simulink model "model_parent_phone"  (R2022a)
settings: Solver=FixedStepAuto  StartTime=0.0  StopTime=inf  RelTol=1e-3
undefined symbols (not defined in the file): Data_Display, Data_Display1, Data_Display2, Data_Display3, map_image, merged
libraries: androiduilib x5, androidcommunicationlib x5, androidaudiovideolib x2
settings Model: Creator=aditya_mangla  LastModifiedBy=aditya_mangla
settings OptimizationCC: EnhancedBackFolding=on  PassReuseOutputArgsAs=Individual arguments  ZeroExternalMemoryAtStartup=off  ZeroInternalMemoryAtStartup=off  MaxStackSize=64  OptimizeBlockOrder=speed  DifferentSizesBufferReuse=on  OptimizationCustomize=off  EfficientTunableParamExpr=on
settings DebuggingCC: ParameterTunabilityLossMsg=error
settings HardwareCC: ProdBitPerPointer=32  ProdBitPerSizeT=32  ProdBitPerPtrDiffT=32  ProdLargestAtomicInteger=Long  ProdLargestAtomicFloat=Double  ProdWordSize=32  ProdHWDeviceType=ARM Compatible->ARM Cortex  UseEmbeddedCoderFeatures=off  UseSimulinkCoderFeatures=off
settings SFSimCC: MATLABDynamicMemAlloc=off
settings RTWCC: SystemTargetFile=ert.tlc  HardwareBoard=Android Device  TLCOptions="-aInlineSetEventsForThisBaseRateFcn=TLC_FALSE -aSuppressMultiTaskScheduler=TLC_FALSE  -aRateBasedStepFcn=0"  TemplateMakefile=ert_default_tmf  RTWVerbose=off  Toolchain=Android SDK/NDK Tools
settings CodeAppCC: ForceParamTrailComments=on  IgnoreCustomStorageClasses=off  OperatorAnnotations=on  SimulinkDataObjDesc=on  SFDataObjDesc=on  InsertBlockDesc=on
settings ERTTargetCC: SupportNonInlinedSFcns=on

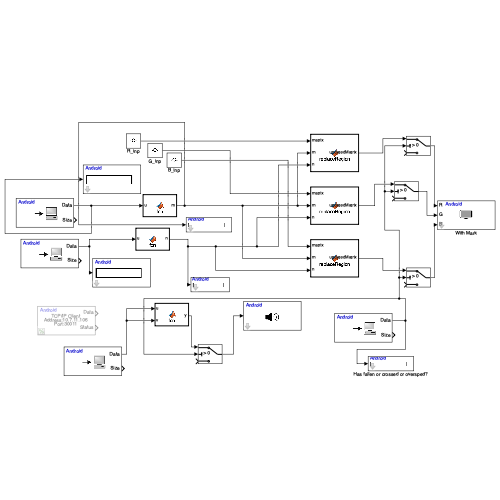
[thumbnail: Simulink's stored preview of the top-level diagram]
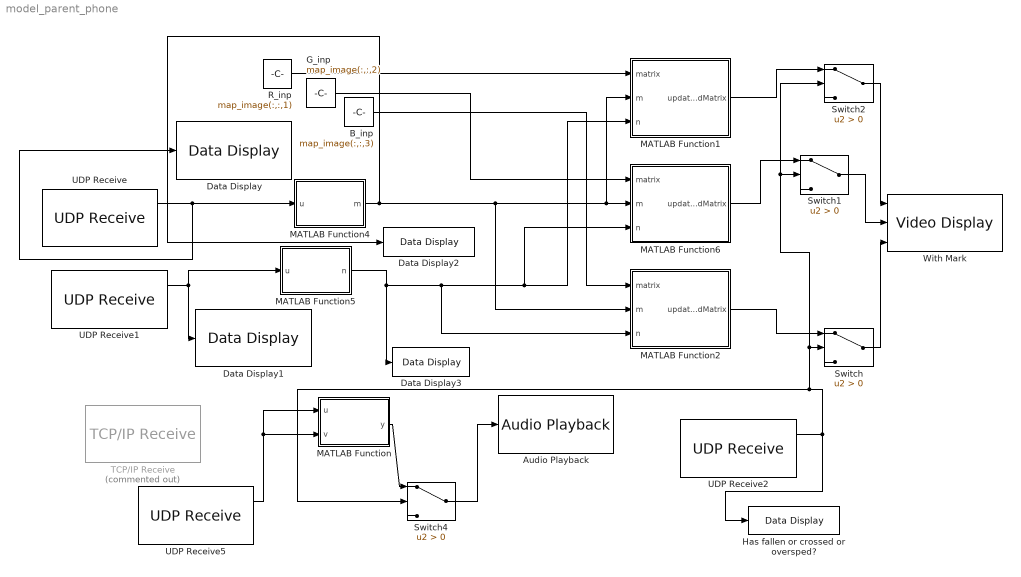
== system model_parent_phone ==
  Audio Playback : androidaudiovideolib/Audio Playback  SampleFreq=24000  AudioSamplingFreq=24000  SampleTime=0.1  DeviceStr=0  QueueDuration=0  BlockPlatform=Android
      settings: SourceProductBaseCode=ANDROID
  B_inp : Constant  Value=map_image(:,:,3)  VectorParams1D=off  OutDataTypeStr=uint8
  Data Display : androiduilib/Data Display  DataDisplayId=merged/Data_Display  Format=Float  Precision=6  SimulateUsing=Code generation  blockPlatform=Android
      settings: SourceProductBaseCode=ANDROID
  Data Display1 : androiduilib/Data Display  DataDisplayId=merged/Data_Display1  Format=Float  Precision=6  SimulateUsing=Code generation  blockPlatform=Android
      settings: SourceProductBaseCode=ANDROID
  Data Display2 : androiduilib/Data Display  DataDisplayId=merged/Data_Display2  Format=Float  Precision=6  SimulateUsing=Code generation  blockPlatform=Android
      settings: SourceProductBaseCode=ANDROID
  Data Display3 : androiduilib/Data Display  DataDisplayId=merged/Data_Display3  Format=Float  Precision=6  SimulateUsing=Code generation  blockPlatform=Android
      settings: SourceProductBaseCode=ANDROID
  G_inp : Constant  Value=map_image(:,:,2)  VectorParams1D=off  OutDataTypeStr=uint8
  Has fallen or crossed or oversped? : androiduilib/Data Display  DataDisplayId=merged/Has_fallen_or_crossed_or_oversped?  Format=Float  Precision=6  SimulateUsing=Code generation  blockPlatform=Android
      settings: SourceProductBaseCode=ANDROID
  MATLAB Function : MATLAB Function  TreatAsAtomicUnit=on
  MATLAB Function1 : MATLAB Function  TreatAsAtomicUnit=on
  MATLAB Function2 : MATLAB Function  TreatAsAtomicUnit=on
  MATLAB Function4 : MATLAB Function  TreatAsAtomicUnit=on
  MATLAB Function5 : MATLAB Function  TreatAsAtomicUnit=on
  MATLAB Function6 : MATLAB Function  TreatAsAtomicUnit=on
  R_inp : Constant  Value=map_image(:,:,1)  VectorParams1D=off  OutDataTypeStr=uint8
  Switch : Switch  Criteria=u2 > Threshold  SaturateOnIntegerOverflow=off  InputSameDT=off
  Switch1 : Switch  Criteria=u2 > Threshold  SaturateOnIntegerOverflow=off  InputSameDT=off
  Switch2 : Switch  Criteria=u2 > Threshold  SaturateOnIntegerOverflow=off  InputSameDT=off
  Switch4 : Switch  Criteria=u2 > Threshold  OutDataTypeStr=int16  SaturateOnIntegerOverflow=off  InputSameDT=off
  TCP/IP Receive : androidcommunicationlib/TCP//IP Receive  Commented=on  TCPReceiveId=Map_display/TCP//IP_Receive  Mode_=Client  LocalServerPort_=25000  RemoteAddr_=10.7.11.106  RemoteServerPort_=30011  DataType_=int16  DataSize_=2400  SampleTime_=0.1  ClientPortBindingSelection_=off  ClientPortToBind_=35000  BlockingMode_=off  BlockTimeout_=0.1
      settings: SourceProductBaseCode=ANDROID
  UDP Receive : androidcommunicationlib/UDP Receive  localURL='0.0.0.0'  localPort=30001  remoteURL='0.0.0.0'  remotePort=-1  recvBufferSize=8192  signalDatatype=double  dims=1  isVarSize=off  showBlockingTime=off  blockingTime=0  sampletime=0.1  blockPlatform=Android
      settings: SourceProductBaseCode=ANDROID
  UDP Receive1 : androidcommunicationlib/UDP Receive  localURL='0.0.0.0'  localPort=30002  remoteURL='0.0.0.0'  remotePort=-1  recvBufferSize=8192  signalDatatype=double  dims=1  isVarSize=off  showBlockingTime=off  blockingTime=0  sampletime=0.1  blockPlatform=Android
      settings: SourceProductBaseCode=ANDROID
  UDP Receive2 : androidcommunicationlib/UDP Receive  localURL='0.0.0.0'  localPort=30012  remoteURL='0.0.0.0'  remotePort=-1  recvBufferSize=8192  signalDatatype=boolean  dims=1  isVarSize=off  showBlockingTime=off  blockingTime=0  sampletime=0.1  blockPlatform=Android
      settings: SourceProductBaseCode=ANDROID
  UDP Receive5 : androidcommunicationlib/UDP Receive  localURL='0.0.0.0'  localPort=30011  remoteURL='0.0.0.0'  remotePort=-1  recvBufferSize=8192  signalDatatype=int16  dims=2400  isVarSize=off  showBlockingTime=off  blockingTime=0  sampletime=0.1  blockPlatform=Android
      settings: SourceProductBaseCode=ANDROID
  With Mark : androidaudiovideolib/Video Display  BlockPlatform=Android
      settings: SourceProductBaseCode=ANDROID
  wires:
  UDP Receive1/1 -> Data Display1/1, MATLAB Function5/1(u)
  Switch4/1 -> Audio Playback/1
  MATLAB Function1/1(updatedMatrix) -> Switch2/1
  MATLAB Function4/1(m) -> Data Display2/1, MATLAB Function1/2(m), MATLAB Function6/2(m), MATLAB Function2/2(m)
  Switch2/1 -> With Mark/1
  B_inp/1 -> MATLAB Function2/1(matrix)
  UDP Receive/1 -> Data Display/1, MATLAB Function4/1(u)
  Switch1/1 -> With Mark/2
  Switch/1 -> With Mark/3
  MATLAB Function6/1(updatedMatrix) -> Switch1/1
  R_inp/1 -> MATLAB Function1/1(matrix)
  MATLAB Function2/1(updatedMatrix) -> Switch/1
  UDP Receive5/1 -> MATLAB Function/2(v), MATLAB Function/1(u)
  G_inp/1 -> MATLAB Function6/1(matrix)
  MATLAB Function/1(y) -> Switch4/1
  MATLAB Function5/1(n) -> Data Display3/1, MATLAB Function1/3(n), MATLAB Function6/3(n), MATLAB Function2/3(n)
  UDP Receive2/1 -> Has fallen or crossed or oversped?/1, Switch4/2, Switch2/2, Switch1/2, Switch/2

== matlab function model_parent_phone/MATLAB Function1 ==
  data: updatedMatrix output; matrix input; m input; n input
function updatedMatrix = replaceRegion(matrix, m, n)
    [rows, cols] = size(matrix);
    updatedMatrix = matrix;


    rowStart = m - 7;
    rowEnd = m + 7;
    colStart = n - 7;
    colEnd = n + 7;

    rowStart = max(1, rowStart);
    rowEnd = min(rows, rowEnd);
    colStart = max(1, colStart);
    colEnd = min(cols, colEnd);

    updatedMatrix(rowStart:rowEnd, colStart:colEnd) = 255; 

end

== matlab function model_parent_phone/MATLAB Function2 ==
  data: updatedMatrix output; matrix input; m input; n input
function updatedMatrix = replaceRegion(matrix, m, n)
    [rows, cols] = size(matrix);
    updatedMatrix = matrix;


    rowStart = m - 7;
    rowEnd = m + 7;
    colStart = n - 7;
    colEnd = n + 7;

    rowStart = max(1, rowStart);
    rowEnd = min(rows, rowEnd);
    colStart = max(1, colStart);
    colEnd = min(cols, colEnd);

    updatedMatrix(rowStart:rowEnd, colStart:colEnd) = 0; 

end

== matlab function model_parent_phone/MATLAB Function4 ==
  data: u input; m output
function m = fcn(u)
    clat=5.513888888888889e-6;
    md = (23.21385-u)/clat;
    m = int16(md);

== matlab function model_parent_phone/MATLAB Function5 ==
  data: u input; n output
function n = fcn(u)
    clong= 3.42890625e-6;
    nd = (72.68525-u)/clong;
    n = int16(nd);

== matlab function model_parent_phone/MATLAB Function ==
  data: u input; y output; v input
function y = fcn(u,v)
    y=[u,v];

end

== matlab function model_parent_phone/MATLAB Function6 ==
  data: updatedMatrix output; matrix input; m input; n input
function updatedMatrix = replaceRegion(matrix, m, n)
    [rows, cols] = size(matrix);
    updatedMatrix = matrix;


    rowStart = m - 7;
    rowEnd = m + 7;
    colStart = n - 7;
    colEnd = n + 7;

    rowStart = max(1, rowStart);
    rowEnd = min(rows, rowEnd);
    colStart = max(1, colStart);
    colEnd = min(cols, colEnd);

    updatedMatrix(rowStart:rowEnd, colStart:colEnd) = 0; 

end
